simulink model "Prev_ThrustTesting"  (R2018a)
settings: Solver=ode4  StartTime=0.0  StopTime=34560000  FixedStep=10  RelTol=1e-3
InitFcn:
  | % Enter your data here
  | 
  | y10 = 152213668;
  | y20 = 0;
  | y30 = 0;
  | y40 = 0;
  | y50 = 34.5845;
  | y60 = 0;
  | y70 = 9700;
settings Model: Creator=jhemi.1  LastModifiedBy=craigheim
settings CodeAppCC: StateflowObjectComments=on

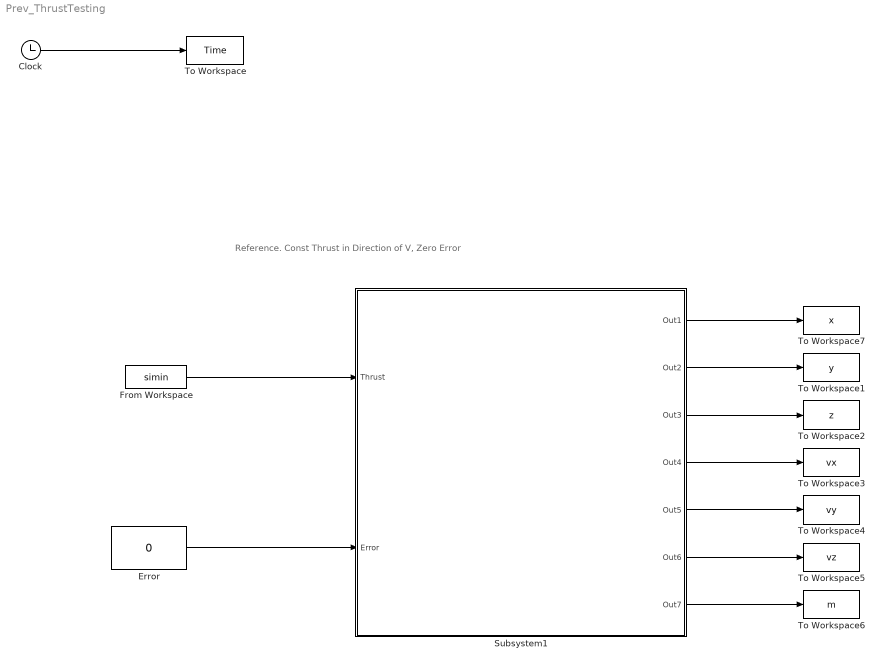
== system Prev_ThrustTesting ==
  note: Reference. Const Thrust in Direction of V, Zero Error
  Clock : Clock
  Error : Constant  Value=0
  From Workspace : FromWorkspace  VariableName=simin  SampleTime=0
  Subsystem1 : Subsystem
  To Workspace : ToWorkspace  VariableName=Time  SampleTime=-1
  To Workspace1 : ToWorkspace  VariableName=y  SampleTime=-1
  To Workspace2 : ToWorkspace  VariableName=z  SampleTime=-1
  To Workspace3 : ToWorkspace  VariableName=vx  SampleTime=-1
  To Workspace4 : ToWorkspace  VariableName=vy  SampleTime=-1
  To Workspace5 : ToWorkspace  VariableName=vz  SampleTime=-1
  To Workspace6 : ToWorkspace  VariableName=m  SampleTime=-1
  To Workspace7 : ToWorkspace  VariableName=x  SampleTime=-1
  wires:
  Clock/1 -> To Workspace/1
  Subsystem1/1(Out1) -> To Workspace7/1
  Subsystem1/2(Out2) -> To Workspace1/1
  Subsystem1/3(Out3) -> To Workspace2/1
  Subsystem1/4(Out4) -> To Workspace3/1
  Subsystem1/5(Out5) -> To Workspace4/1
  Subsystem1/6(Out6) -> To Workspace5/1
  Subsystem1/7(Out7) -> To Workspace6/1
  Error/1 -> Subsystem1/2(Error)
  From Workspace/1 -> Subsystem1/1(Thrust)

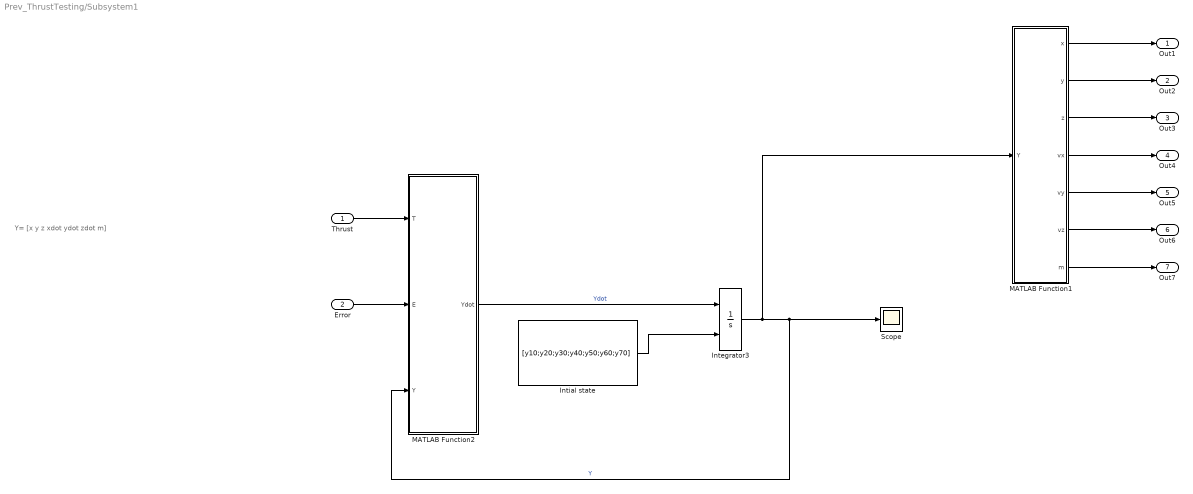
== system Prev_ThrustTesting/Subsystem1 ==
  note: Y= [x
      | y
      | z
      | xdot
      | ydot
      | zdot
      | m]
  Thrust : Inport
  Error : Inport  Port=2
  Integrator3 : Integrator  InitialConditionSource=external
  Intial state : Constant  Value=[y10;y20;y30;y40;y50;y60;y70]
  MATLAB Function1 : MATLAB Function  TreatAsAtomicUnit=on
  MATLAB Function2 : MATLAB Function  TreatAsAtomicUnit=on
  Scope : Scope
  Out1 : Outport
  Out2 : Outport  Port=2
  Out3 : Outport  Port=3
  Out4 : Outport  Port=4
  Out5 : Outport  Port=5
  Out6 : Outport  Port=6
  Out7 : Outport  Port=7
  wires:
  MATLAB Function1/1(x) -> Out1/1
  MATLAB Function2/1(Ydot) -> Integrator3/1  "Ydot"
  MATLAB Function1/5(vy) -> Out5/1
  Thrust/1 -> MATLAB Function2/1(T)
  MATLAB Function1/4(vx) -> Out4/1
  Integrator3/1 -> MATLAB Function1/1(Y), MATLAB Function2/3(Y), Scope/1  "Y"
  MATLAB Function1/6(vz) -> Out6/1
  MATLAB Function1/3(z) -> Out3/1
  MATLAB Function1/2(y) -> Out2/1
  Intial state/1 -> Integrator3/2
  MATLAB Function1/7(m) -> Out7/1
  Error/1 -> MATLAB Function2/2(E)

== matlab function Prev_ThrustTesting/Subsystem1/MATLAB Function1 ==
  data: x output; y output; z output; vx output; vy output; vz output; Y input; m output
function [x,y,z,vx,vy,vz,m] = fcn(Y)
% This function does ......,.
%
% constants
 

% reading the OED variable from Y
x = Y(1);  % x
y = Y(2);  % y
z = Y(3);  % z
vx = Y(4);  % xdot
vy = Y(5);  % ydot
vz = Y(6);  % zdot
m  = Y(7);  % m



 
% end of function

== matlab function Prev_ThrustTesting/Subsystem1/MATLAB Function2 ==
  data: T input; E input; Y input; Ydot output
function Ydot = fcn(T,E,Y)
% This function does ......,.
% T = thrust [N]
% E = error/noise

% constants
Isp = 850;
g0 = 9.81*10^-3;
mu = 1.3275*10^11;

% reading the OED variable from Y
y1 = Y(1);  % x
y2 = Y(2);  % y
y3 = Y(3);  % z
y4 = Y(4);  % xdot
y5 = Y(5);  % ydot
y6 = Y(6);  % zdot
m  = Y(7);  % m

% Computing velocity, position 
V = sqrt(y4^2+y5^2+y6^2); % velocity
r = sqrt(y1^2+y2^2+y3^2); % position
%
% Computing Ydot (ODE implemnetation)
Ydot = [y4;
        y5;
        y6;
       -mu*y1/r^3 + T/m*y4/V + E;   
       -mu*y2/r^3 + T/m*y5/V + E;
       -mu*y3/r^3 + T/m*y6/V + E;
       -abs(T)/(Isp*g0)
       ];
% end of function
